simulink model "P4_disturbance_sim"  (R2021b)
settings: Solver=VariableStepAuto  StartTime=0.0  StopTime=Tmax  RelTol=1e-3
values from neighbouring files (symbols this model uses):
  a = g/L    (= 32.6666666667)    [P4_1.m]    (also in P4_2_1.m; P4_2_2.m; P4_2_3.m; P4_3.m)
  b = k/m    (= 0.1)    [P4_1.m]    (also in P4_2_1.m; P4_2_2.m; P4_2_3.m; P4_3.m)
  c = 1/(m*L^2)    (= 111.111111111)    [P4_1.m]    (also in P4_2_1.m; P4_2_2.m; P4_2_3.m; P4_3.m)
  h = 0.1    [P4_1.m]    (also in P4_2_1.m; P4_2_2.m; P4_2_3.m; P4_3.m)
  md = MPCInit(Ad,Bd,Cyd,Czd,Dzd,Ccd,Dcd,Hp,Hw,zblk,Hu,ublk,  	    du_max,du_min,u_max,u_min,z_max,  	    z_min,Q,R,W,V,h,cmode,solver)    [P4_1.m]    (also in P4_2_1.m = MPCInit(Ad,Bd,Cyd,Czd,Dzd,Ccd,Dcd,Hp,Hw,zblk,Hu,ublk,  	    ; P4_2_2.m = MPCInit(Ad,Bd,Cyd,Czd,Dzd,Ccd,Dcd,Hp,Hw,zblk,Hu,ublk,  	    ; P4_2_3.m = MPCInit(Ad,Bd,Cyd,Czd,Dzd,Ccd,Dcd,Hp,Hw,zblk,Hu,ublk,  	    ; P4_3.m = MPCInit(Ad,Bd,Cyd,Czd,Dzd,Ccd,Dcd,Hp,Hw,zblk,Hu,ublk,  	    )
  ref_amp = 15 * pi/180    (= 0.261799387799)    [P4_1.m]    (also in P4_2_1.m = 0; P4_2_2.m = 0.174532925199; P4_2_3.m = 0; P4_3.m = 0)
  ref_step_start = 0.5    [P4_1.m]    (also in P4_2_1.m = 0; P4_2_2.m = 2; P4_2_3.m = 0; P4_3.m = 0)
  ref_step_time = 11    [P4_1.m]    (also in P4_2_1.m; P4_2_2.m; P4_2_3.m; P4_3.m)
  theta0 = 0 * pi/180    (= 0)    [P4_1.m]    (also in P4_2_1.m = 0.523598775598; P4_2_2.m; P4_2_3.m = 0.523598775598; P4_3.m = theta0_vector(i))
undefined symbols (not defined in the file or in its folder): ref_freq
settings Model: Creator=User  LastModifiedBy=User
settings DataIOCC: ReturnWorkspaceOutputs=off

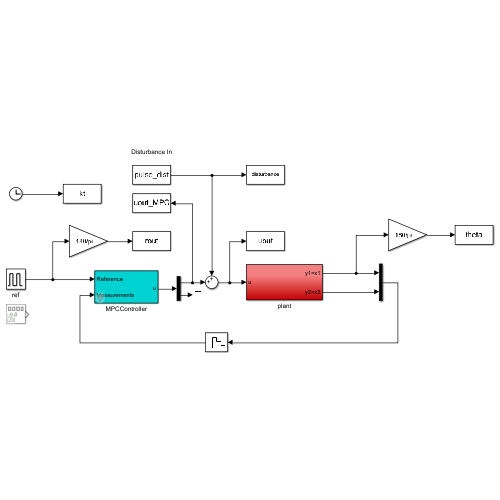
[thumbnail: Simulink's stored preview of the top-level diagram]
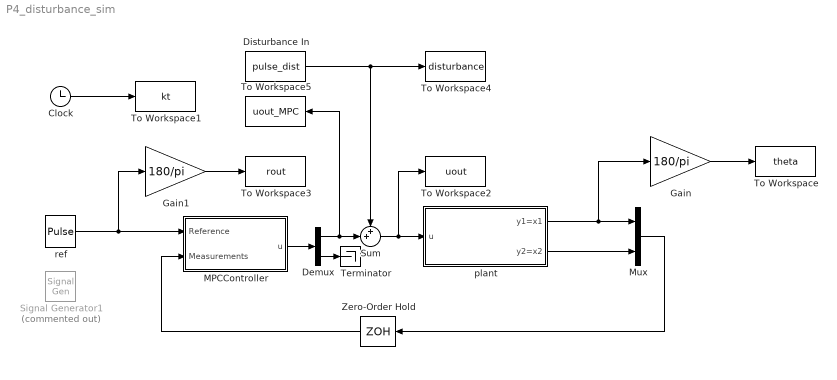
== system P4_disturbance_sim ==
  Clock : Clock
  Demux : Demux  Outputs=[md.m md.ne]
      settings: DisplayOption=none
  "Disturbance In " : FromWorkspace  VariableName=pulse_dist  SampleTime=h
  Gain : Gain  Gain=180/pi
  Gain1 : Gain  Gain=180/pi
  MPCController : Subsystem  mask{md=md}
      mask prompts: md "MPCData"
  Mux : Mux  Inputs=2
  Signal Generator1 : SignalGenerator  Commented=on  WaveForm=square  Amplitude=ref_amp  Frequency=ref_freq
  Sum : Sum  Inputs=++|
  Terminator : Terminator
  To Workspace : ToWorkspace  VariableName=theta  SampleTime=-1
  To Workspace1 : ToWorkspace  VariableName=kt  SampleTime=-1
  To Workspace2 : ToWorkspace  VariableName=uout  SaveFormat=Structure With Time  SampleTime=-1
  To Workspace3 : ToWorkspace  VariableName=rout  SampleTime=-1
  To Workspace4 : ToWorkspace  VariableName=disturbance  SaveFormat=Structure With Time  SampleTime=-1
  To Workspace5 : ToWorkspace  VariableName=uout_MPC  SaveFormat=Structure With Time  SampleTime=-1
  Zero-Order Hold : ZeroOrderHold  SampleTime=h
  plant : Subsystem
  ref : DiscretePulseGenerator  PulseType=Time based  Amplitude=ref_amp  Period=100  PulseWidth=ref_step_time  PhaseDelay=ref_step_start
  wires:
  Gain1/1 -> To Workspace3/1
  Mux/1 -> Zero-Order Hold/1
  Demux/2 -> Terminator/1
  plant/1(y1=x1) -> Mux/1, Gain/1
  ref/1 -> Gain1/1, MPCController/1(Reference)
  plant/2(y2=x2) -> Mux/2
  Zero-Order Hold/1 -> MPCController/2(Measurements)
  MPCController/1(u) -> Demux/1
  Gain/1 -> To Workspace/1
  Clock/1 -> To Workspace1/1
  Demux/1 -> To Workspace5/1, Sum/2
  Sum/1 -> To Workspace2/1, plant/1(u)
  "Disturbance In "/1 -> To Workspace4/1, Sum/1

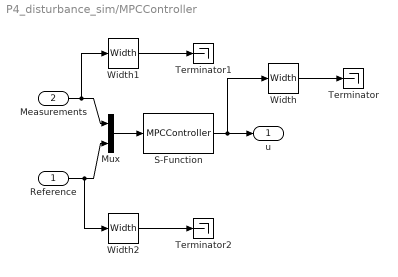
== system P4_disturbance_sim/MPCController ==
  Reference : Inport
  Measurements : Inport  Port=2
  Mux : Mux  Inputs=2
  S-Function : S-Function  FunctionName=MPCController  Parameters=md  SFunctionDeploymentMode=off  EnableBusSupport=off
  Terminator : Terminator
  Terminator1 : Terminator
  Terminator2 : Terminator
  Width : Width
  Width1 : Width
  Width2 : Width
  u : Outport  VectorParamsAs1DForOutWhenUnconnected=off
  wires:
  Mux/1 -> S-Function/1
  Measurements/1 -> Width1/1, Mux/1
  Reference/1 -> Width2/1, Mux/2
  S-Function/1 -> Width/1, u/1
  Width/1 -> Terminator/1
  Width1/1 -> Terminator1/1
  Width2/1 -> Terminator2/1

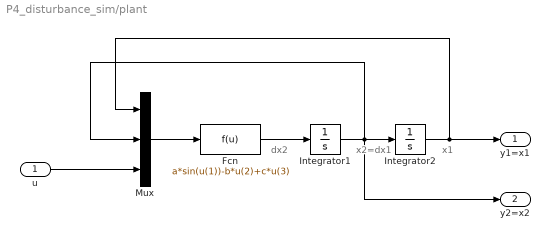
== system P4_disturbance_sim/plant ==
  note: x2=dx1
  note: dx2
  note: x1
  u : Inport
  Fcn : Fcn  Expr=a*sin(u(1))-b*u(2)+c*u(3)
  "Integrator1 " : Integrator
  "Integrator2 " : Integrator  InitialCondition=theta0
  Mux : Mux  Inputs=3
  y1=x1 : Outport  VectorParamsAs1DForOutWhenUnconnected=off
  y2=x2 : Outport  Port=2  VectorParamsAs1DForOutWhenUnconnected=off
  wires:
  u/1 -> Mux/3
  Mux/1 -> Fcn/1
  "Integrator1 "/1 -> y2=x2/1, Mux/2, "Integrator2 "/1
  Fcn/1 -> "Integrator1 "/1
  "Integrator2 "/1 -> y1=x1/1, Mux/1
